simulink model "PlantWrapper"  (R2026a)
settings: Solver=FixedStepAuto  StopTime=100
undefined symbols (not defined in the file): DiscIntNeverNeededParam, simulationParams
settings Model: Creator=rayyu  LastModifiedBy=rayyu

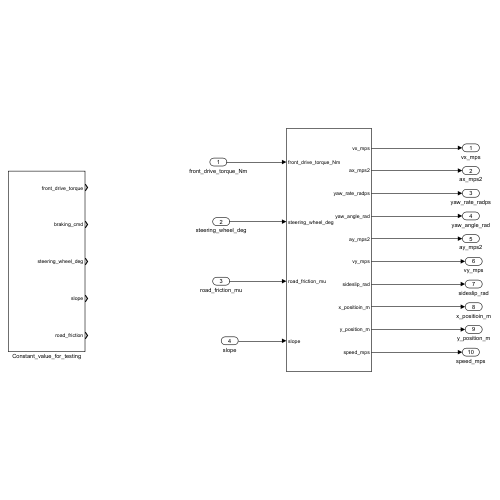
[thumbnail: Simulink's stored preview of the top-level diagram]
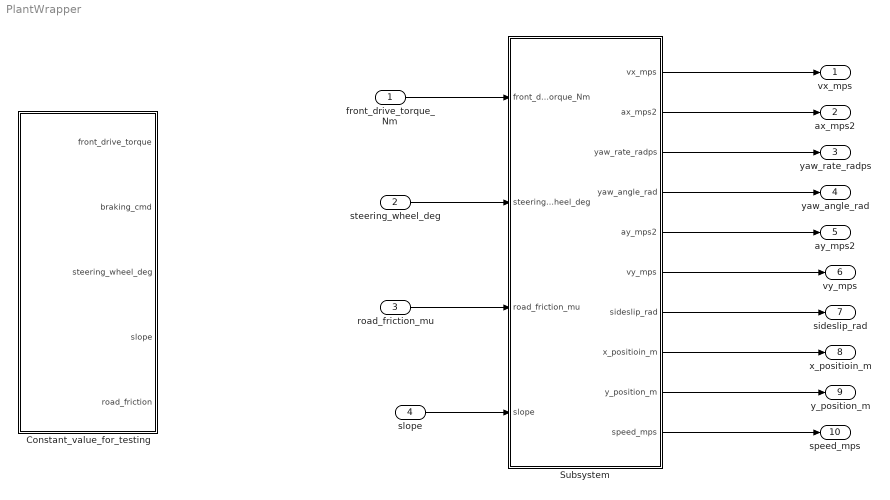
== system PlantWrapper ==
  front_drive_torque_Nm : Inport
  steering_wheel_deg : Inport  Port=2
  road_friction_mu : Inport  Port=3
  slope : Inport  Port=4
  Constant_value_for_testing : Subsystem
  Subsystem : Subsystem
  vx_mps : Outport
  ax_mps2 : Outport  Port=2
  yaw_rate_radps : Outport  Port=3
  yaw_angle_rad : Outport  Port=4
  ay_mps2 : Outport  Port=5
  vy_mps : Outport  Port=6
  sideslip_rad : Outport  Port=7
  x_positioin_m : Outport  Port=8
  y_position_m : Outport  Port=9
  speed_mps : Outport  Port=10
  wires:
  Subsystem/1(vx_mps) -> vx_mps/1
  Subsystem/2(ax_mps2) -> ax_mps2/1
  Subsystem/3(yaw_rate_radps) -> yaw_rate_radps/1
  Subsystem/4(yaw_angle_rad) -> yaw_angle_rad/1
  Subsystem/5(ay_mps2) -> ay_mps2/1
  Subsystem/6(vy_mps) -> vy_mps/1
  Subsystem/7(sideslip_rad) -> sideslip_rad/1
  road_friction_mu/1 -> Subsystem/3(road_friction_mu)
  steering_wheel_deg/1 -> Subsystem/2(steering_wheel_deg)
  front_drive_torque_Nm/1 -> Subsystem/1(front_drive_torque_Nm)
  Subsystem/8(x_positioin_m) -> x_positioin_m/1
  Subsystem/9(y_position_m) -> y_position_m/1
  Subsystem/10(speed_mps) -> speed_mps/1
  slope/1 -> Subsystem/4(slope)

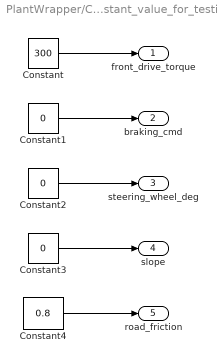
== system PlantWrapper/Constant_value_for_testing ==
  Constant : Constant  Value=300
  Constant1 : Constant  Value=0
  Constant2 : Constant  Value=0
  Constant3 : Constant  Value=0
  Constant4 : Constant  Value=0.8
  front_drive_torque : Outport
  braking_cmd : Outport  Port=2
  steering_wheel_deg : Outport  Port=3
  slope : Outport  Port=4
  road_friction : Outport  Port=5
  wires:
  Constant1/1 -> braking_cmd/1
  Constant4/1 -> road_friction/1
  Constant2/1 -> steering_wheel_deg/1
  Constant3/1 -> slope/1
  Constant/1 -> front_drive_torque/1

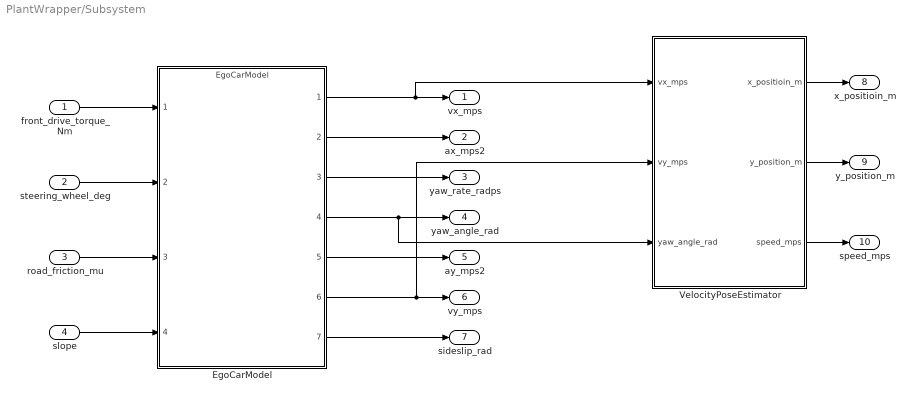
== system PlantWrapper/Subsystem ==
  front_drive_torque_Nm : Inport
  steering_wheel_deg : Inport  Port=2
  road_friction_mu : Inport  Port=3
  slope : Inport  Port=4
  EgoCarModel : ModelReference  ModelNameDialog=EgoCarModel.slx  SimulationMode=Normal  ModelReferenceVersion=1.32
  VelocityPoseEstimator : Subsystem
  vx_mps : Outport
  ax_mps2 : Outport  Port=2
  yaw_rate_radps : Outport  Port=3
  yaw_angle_rad : Outport  Port=4
  ay_mps2 : Outport  Port=5
  vy_mps : Outport  Port=6
  sideslip_rad : Outport  Port=7
  x_positioin_m : Outport  Port=8
  y_position_m : Outport  Port=9
  speed_mps : Outport  Port=10
  wires:
  front_drive_torque_Nm/1 -> EgoCarModel/1
  EgoCarModel/1 -> VelocityPoseEstimator/1(vx_mps), vx_mps/1
  road_friction_mu/1 -> EgoCarModel/3
  EgoCarModel/2 -> ax_mps2/1
  EgoCarModel/3 -> yaw_rate_radps/1
  EgoCarModel/4 -> VelocityPoseEstimator/3(yaw_angle_rad), yaw_angle_rad/1
  EgoCarModel/5 -> ay_mps2/1
  EgoCarModel/6 -> VelocityPoseEstimator/2(vy_mps), vy_mps/1
  EgoCarModel/7 -> sideslip_rad/1
  VelocityPoseEstimator/1(x_positioin_m) -> x_positioin_m/1
  VelocityPoseEstimator/2(y_position_m) -> y_position_m/1
  VelocityPoseEstimator/3(speed_mps) -> speed_mps/1
  steering_wheel_deg/1 -> EgoCarModel/2
  slope/1 -> EgoCarModel/4

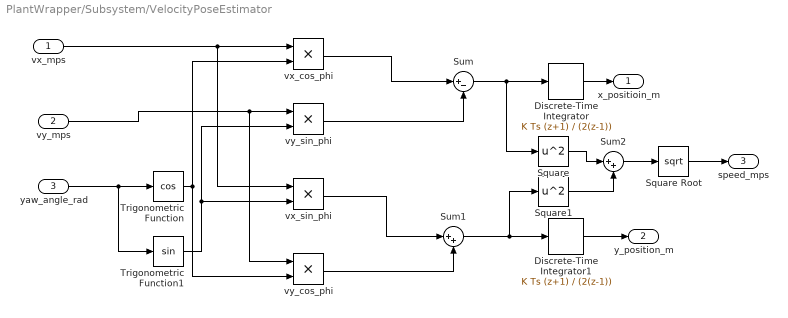
== system PlantWrapper/Subsystem/VelocityPoseEstimator ==
  vx_mps : Inport
  vy_mps : Inport  Port=2
  yaw_angle_rad : Inport  Port=3
  Discrete-Time Integrator : DiscreteIntegrator  IntegratorMethod=Integration: Trapezoidal  InitialCondition=simulationParams.initial_x_m  SampleTime=simulationParams.plant_step_s  ICPrevOutput=DiscIntNeverNeededParam  ICPrevScaledInput=DiscIntNeverNeededParam
  Discrete-Time Integrator1 : DiscreteIntegrator  IntegratorMethod=Integration: Trapezoidal  InitialCondition=simulationParams.initial_y_m  SampleTime=simulationParams.plant_step_s  ICPrevOutput=DiscIntNeverNeededParam  ICPrevScaledInput=DiscIntNeverNeededParam
  Square : Math  Operator=square
  Square Root : Sqrt
  Square1 : Math  Operator=square
  Sum : Sum  Inputs=|+-
  Sum1 : Sum  Inputs=|++
  Sum2 : Sum  Inputs=|++
  Trigonometric Function : Trigonometry  Operator=cos
  Trigonometric Function1 : Trigonometry
  vx_cos_phi : Product
  vx_sin_phi : Product
  vy_cos_phi : Product
  vy_sin_phi : Product
  x_positioin_m : Outport
  y_position_m : Outport  Port=2
  speed_mps : Outport  Port=3
  wires:
  yaw_angle_rad/1 -> Trigonometric Function1/1, Trigonometric Function/1
  vx_mps/1 -> vx_sin_phi/1, vx_cos_phi/1
  Trigonometric Function/1 -> vx_cos_phi/2, vy_cos_phi/2
  vy_mps/1 -> vy_cos_phi/1, vy_sin_phi/1
  Trigonometric Function1/1 -> vy_sin_phi/2, vx_sin_phi/2
  vx_cos_phi/1 -> Sum/1
  vy_sin_phi/1 -> Sum/2
  vx_sin_phi/1 -> Sum1/1
  vy_cos_phi/1 -> Sum1/2
  Sum/1 -> Square/1, Discrete-Time Integrator/1
  Sum1/1 -> Square1/1, Discrete-Time Integrator1/1
  Discrete-Time Integrator/1 -> x_positioin_m/1
  Discrete-Time Integrator1/1 -> y_position_m/1
  Square/1 -> Sum2/1
  Square1/1 -> Sum2/2
  Sum2/1 -> Square Root/1
  Square Root/1 -> speed_mps/1
